simulink model "case1"  (R2024b)
settings: Solver=FixedStepAuto  StartTime=0  StopTime=1  FixedStep=1e-7  RelTol=1e-3
values from neighbouring files (symbols this model uses):
  SG_D_1_D = 0.01056    [IEEE9_case_parameters.m]    (also in case1_parameters.m; case2_parameters.m; case3_parameters.m; case4_parameters.m)
  SG_D_1_EnableSaturation = 0    [IEEE9_case_parameters.m]    (also in case1_parameters.m; case2_parameters.m; case3_parameters.m; case4_parameters.m)
  SG_D_1_f0 = 60    [IEEE9_case_parameters.m]    (also in case1_parameters.m; case2_parameters.m; case3_parameters.m; case4_parameters.m)
  SG_D_1_H = 7.5    [IEEE9_case_parameters.m]    (also in case1_parameters.m; case2_parameters.m; case3_parameters.m; case4_parameters.m)
  SG_D_1_K_A = 20    [IEEE9_case_parameters.m]    (also in case1_parameters.m; case2_parameters.m; case3_parameters.m; case4_parameters.m)
  SG_D_1_K_E = 1.000000e+1    (= 10)    [IEEE9_case_parameters.m]    (also in case1_parameters.m; case2_parameters.m; case3_parameters.m; case4_parameters.m)
  SG_D_1_K_F = 2.363    [IEEE9_case_parameters.m]    (also in case1_parameters.m; case2_parameters.m; case3_parameters.m; case4_parameters.m)
  SG_D_1_K_s = 0.5    [IEEE9_case_parameters.m]    (also in case1_parameters.m = 5; case2_parameters.m = 5; case3_parameters.m = 5; case4_parameters.m = 5)
  SG_D_1_R_a = 0.001088    [IEEE9_case_parameters.m]    (also in case1_parameters.m; case2_parameters.m; case3_parameters.m; case4_parameters.m)
  SG_D_1_S_A = 1    [IEEE9_case_parameters.m]    (also in case1_parameters.m; case2_parameters.m; case3_parameters.m; case4_parameters.m)
  SG_D_1_S_B = 0.103    [IEEE9_case_parameters.m]    (also in case1_parameters.m; case2_parameters.m; case3_parameters.m; case4_parameters.m)
  SG_D_1_S_N = 10.659857    [IEEE9_case_parameters.m]    (also in case1_parameters.m; case2_parameters.m; case3_parameters.m; case4_parameters.m)
  SG_D_1_SpeedPara = 200    [IEEE9_case_parameters.m]    (also in case1_parameters.m; case2_parameters.m; case3_parameters.m; case4_parameters.m)
  SG_D_1_T_0 = 0.720173    [IEEE9_case_parameters.m]    (also in case1_parameters.m = 0.755522; case2_parameters.m = 0.808931; case3_parameters.m = 0.869402; case4_parameters.m = 0.729316)
  SG_D_1_T_1 = 0.3    [IEEE9_case_parameters.m]    (also in case1_parameters.m; case2_parameters.m; case3_parameters.m; case4_parameters.m)
  SG_D_1_T_2 = 0.05    [IEEE9_case_parameters.m]    (also in case1_parameters.m; case2_parameters.m; case3_parameters.m; case4_parameters.m)
  SG_D_1_T_3 = 0.02    [IEEE9_case_parameters.m]    (also in case1_parameters.m; case2_parameters.m; case3_parameters.m; case4_parameters.m)
  SG_D_1_T_4 = 0.005    [IEEE9_case_parameters.m]    (also in case1_parameters.m; case2_parameters.m; case3_parameters.m; case4_parameters.m)
  SG_D_1_T_A = 0.02    [IEEE9_case_parameters.m]    (also in case1_parameters.m; case2_parameters.m; case3_parameters.m; case4_parameters.m)
  SG_D_1_T_dd = 8.000000e+0    (= 8)    [IEEE9_case_parameters.m]    (also in case1_parameters.m; case2_parameters.m; case3_parameters.m; case4_parameters.m)
  SG_D_1_T_ddd = 0.04    [IEEE9_case_parameters.m]    (also in case1_parameters.m; case2_parameters.m; case3_parameters.m; case4_parameters.m)
  SG_D_1_T_E = 0.314    [IEEE9_case_parameters.m]    (also in case1_parameters.m; case2_parameters.m; case3_parameters.m; case4_parameters.m)
  SG_D_1_T_F = 0.35    [IEEE9_case_parameters.m]    (also in case1_parameters.m; case2_parameters.m; case3_parameters.m; case4_parameters.m)
  SG_D_1_T_qd = 0.8    [IEEE9_case_parameters.m]    (also in case1_parameters.m; case2_parameters.m; case3_parameters.m; case4_parameters.m)
  SG_D_1_T_qdd = 0.02    [IEEE9_case_parameters.m]    (also in case1_parameters.m; case2_parameters.m; case3_parameters.m; case4_parameters.m)
  SG_D_1_T_speed = 0.1    [IEEE9_case_parameters.m]    (also in case1_parameters.m = 200; case2_parameters.m = 200; case3_parameters.m = 200; case4_parameters.m = 200)
  SG_D_1_T_w = 0.5    [IEEE9_case_parameters.m]    (also in case1_parameters.m; case2_parameters.m; case3_parameters.m; case4_parameters.m)
  SG_D_1_V_ref = 1.990276    [IEEE9_case_parameters.m]    (also in case1_parameters.m = 2.042296; case2_parameters.m = 2.051388; case3_parameters.m = 2.089584; case4_parameters.m = 2.01845)
  SG_D_1_w_ref = 376.991118    [IEEE9_case_parameters.m]    (also in case1_parameters.m; case2_parameters.m; case3_parameters.m; case4_parameters.m)
  SG_D_1_wb = 6.000000e+1    (= 60)    [IEEE9_case_parameters.m]    (also in case1_parameters.m; case2_parameters.m; case3_parameters.m; case4_parameters.m)
  SG_D_1_x_d = 1.9    [IEEE9_case_parameters.m]    (also in case1_parameters.m; case2_parameters.m; case3_parameters.m; case4_parameters.m)
  SG_D_1_x_dd = 0.302    [IEEE9_case_parameters.m]    (also in case1_parameters.m; case2_parameters.m; case3_parameters.m; case4_parameters.m)
  SG_D_1_x_ddd = 0.204    [IEEE9_case_parameters.m]    (also in case1_parameters.m; case2_parameters.m; case3_parameters.m; case4_parameters.m)
  SG_D_1_x_l = 0.05    [IEEE9_case_parameters.m]    (also in case1_parameters.m; case2_parameters.m; case3_parameters.m; case4_parameters.m)
  SG_D_1_x_q = 1.3    [IEEE9_case_parameters.m]    (also in case1_parameters.m; case2_parameters.m; case3_parameters.m; case4_parameters.m)
  SG_D_1_x_qd = 0.5    [IEEE9_case_parameters.m]    (also in case1_parameters.m; case2_parameters.m; case3_parameters.m; case4_parameters.m)
  SG_D_1_x_qdd = 0.3    [IEEE9_case_parameters.m]    (also in case1_parameters.m; case2_parameters.m; case3_parameters.m; case4_parameters.m)
  SG_D_2_D = 0.02    [IEEE9_case_parameters.m]    (also in case1_parameters.m; case2_parameters.m; case3_parameters.m; case4_parameters.m)
  SG_D_2_EnableSaturation = 0    [IEEE9_case_parameters.m]    (also in case1_parameters.m; case2_parameters.m; case3_parameters.m; case4_parameters.m)
  SG_D_2_f0 = 60    [IEEE9_case_parameters.m]    (also in case1_parameters.m; case2_parameters.m; case3_parameters.m; case4_parameters.m)
  SG_D_2_H = 8.000000e+0    (= 8)    [IEEE9_case_parameters.m]    (also in case1_parameters.m; case2_parameters.m; case3_parameters.m; case4_parameters.m)
  SG_D_2_K_A = 20    [IEEE9_case_parameters.m]    (also in case1_parameters.m; case2_parameters.m; case3_parameters.m; case4_parameters.m)
  SG_D_2_K_E = 1.000000e+1    (= 10)    [IEEE9_case_parameters.m]    (also in case1_parameters.m; case2_parameters.m; case3_parameters.m; case4_parameters.m)
  SG_D_2_K_F = 2.363    [IEEE9_case_parameters.m]    (also in case1_parameters.m; case2_parameters.m; case3_parameters.m; case4_parameters.m)
  SG_D_2_K_s = 0.5    [IEEE9_case_parameters.m]    (also in case1_parameters.m = 4; case2_parameters.m = 4; case3_parameters.m = 4; case4_parameters.m = 4)
  SG_D_2_R_a = 0.001088    [IEEE9_case_parameters.m]    (also in case1_parameters.m; case2_parameters.m; case3_parameters.m; case4_parameters.m)
  SG_D_2_S_A = 1    [IEEE9_case_parameters.m]    (also in case1_parameters.m; case2_parameters.m; case3_parameters.m; case4_parameters.m)
  SG_D_2_S_B = 0.103    [IEEE9_case_parameters.m]    (also in case1_parameters.m; case2_parameters.m; case3_parameters.m; case4_parameters.m)
  SG_D_2_S_N = 10.659857    [IEEE9_case_parameters.m]    (also in case1_parameters.m; case2_parameters.m; case3_parameters.m; case4_parameters.m)
  SG_D_2_SpeedPara = 200    [IEEE9_case_parameters.m]    (also in case1_parameters.m; case2_parameters.m; case3_parameters.m; case4_parameters.m)
  SG_D_2_T_0 = 1.632913    [IEEE9_case_parameters.m]    (also in case1_parameters.m = 1.632925; case2_parameters.m = 1.632915; case3_parameters.m = 1.632914; case4_parameters.m = 1.632927)
  SG_D_2_T_1 = 0.2    [IEEE9_case_parameters.m]    (also in case1_parameters.m; case2_parameters.m; case3_parameters.m; case4_parameters.m)
  SG_D_2_T_2 = 0.05    [IEEE9_case_parameters.m]    (also in case1_parameters.m; case2_parameters.m; case3_parameters.m; case4_parameters.m)
  SG_D_2_T_3 = 0.02    [IEEE9_case_parameters.m]    (also in case1_parameters.m; case2_parameters.m; case3_parameters.m; case4_parameters.m)
  SG_D_2_T_4 = 0.005    [IEEE9_case_parameters.m]    (also in case1_parameters.m; case2_parameters.m; case3_parameters.m; case4_parameters.m)
  SG_D_2_T_A = 0.02    [IEEE9_case_parameters.m]    (also in case1_parameters.m; case2_parameters.m; case3_parameters.m; case4_parameters.m)
  SG_D_2_T_dd = 7.9    [IEEE9_case_parameters.m]    (also in case1_parameters.m; case2_parameters.m; case3_parameters.m; case4_parameters.m)
  SG_D_2_T_ddd = 0.04    [IEEE9_case_parameters.m]    (also in case1_parameters.m; case2_parameters.m; case3_parameters.m; case4_parameters.m)
  SG_D_2_T_E = 0.314    [IEEE9_case_parameters.m]    (also in case1_parameters.m; case2_parameters.m; case3_parameters.m; case4_parameters.m)
  SG_D_2_T_F = 0.35    [IEEE9_case_parameters.m]    (also in case1_parameters.m; case2_parameters.m; case3_parameters.m; case4_parameters.m)
  SG_D_2_T_qd = 0.8    [IEEE9_case_parameters.m]    (also in case1_parameters.m; case2_parameters.m; case3_parameters.m; case4_parameters.m)
  SG_D_2_T_qdd = 0.015    [IEEE9_case_parameters.m]    (also in case1_parameters.m; case2_parameters.m; case3_parameters.m; case4_parameters.m)
  SG_D_2_T_speed = 0.1    [IEEE9_case_parameters.m]    (also in case1_parameters.m = 150; case2_parameters.m = 150; case3_parameters.m = 150; case4_parameters.m = 150)
  SG_D_2_T_w = 0.35    [IEEE9_case_parameters.m]    (also in case1_parameters.m; case2_parameters.m; case3_parameters.m; case4_parameters.m)
  SG_D_2_V_ref = 2.58547    [IEEE9_case_parameters.m]    (also in case1_parameters.m = 2.597896; case2_parameters.m = 2.587136; case3_parameters.m = 2.586042; case4_parameters.m = 2.599679)
  SG_D_2_w_ref = 376.991118    [IEEE9_case_parameters.m]    (also in case1_parameters.m; case2_parameters.m; case3_parameters.m; case4_parameters.m)
  SG_D_2_wb = 6.000000e+1    (= 60)    [IEEE9_case_parameters.m]    (also in case1_parameters.m; case2_parameters.m; case3_parameters.m; case4_parameters.m)
  SG_D_2_x_d = 1.8    [IEEE9_case_parameters.m]    (also in case1_parameters.m; case2_parameters.m; case3_parameters.m; case4_parameters.m)
  SG_D_2_x_dd = 0.302    [IEEE9_case_parameters.m]    (also in case1_parameters.m; case2_parameters.m; case3_parameters.m; case4_parameters.m)
  SG_D_2_x_ddd = 0.204    [IEEE9_case_parameters.m]    (also in case1_parameters.m; case2_parameters.m; case3_parameters.m; case4_parameters.m)
  SG_D_2_x_l = 0.05    [IEEE9_case_parameters.m]    (also in case1_parameters.m; case2_parameters.m; case3_parameters.m; case4_parameters.m)
  SG_D_2_x_q = 1.25    [IEEE9_case_parameters.m]    (also in case1_parameters.m; case2_parameters.m; case3_parameters.m; case4_parameters.m)
  SG_D_2_x_qd = 0.5    [IEEE9_case_parameters.m]    (also in case1_parameters.m; case2_parameters.m; case3_parameters.m; case4_parameters.m)
  SG_D_2_x_qdd = 0.3    [IEEE9_case_parameters.m]    (also in case1_parameters.m; case2_parameters.m; case3_parameters.m; case4_parameters.m)
  SG_D_3_D = 0.02    [IEEE9_case_parameters.m]    (also in case1_parameters.m; case2_parameters.m; case3_parameters.m; case4_parameters.m)
  SG_D_3_EnableSaturation = 0    [IEEE9_case_parameters.m]    (also in case1_parameters.m; case2_parameters.m; case3_parameters.m; case4_parameters.m)
  SG_D_3_f0 = 60    [IEEE9_case_parameters.m]    (also in case1_parameters.m; case2_parameters.m; case3_parameters.m; case4_parameters.m)
  SG_D_3_H = 7.7    [IEEE9_case_parameters.m]    (also in case1_parameters.m; case2_parameters.m; case3_parameters.m; case4_parameters.m)
  SG_D_3_K_A = 20    [IEEE9_case_parameters.m]    (also in case1_parameters.m; case2_parameters.m; case3_parameters.m; case4_parameters.m)
  SG_D_3_K_E = 1.000000e+1    (= 10)    [IEEE9_case_parameters.m]    (also in case1_parameters.m; case2_parameters.m; case3_parameters.m; case4_parameters.m)
  SG_D_3_K_F = 2.363    [IEEE9_case_parameters.m]    (also in case1_parameters.m; case2_parameters.m; case3_parameters.m; case4_parameters.m)
  SG_D_3_K_s = 0.2    [IEEE9_case_parameters.m]    (also in case1_parameters.m = 2; case2_parameters.m = 2; case3_parameters.m = 2; case4_parameters.m = 2)
  SG_D_3_R_a = 0.001088    [IEEE9_case_parameters.m]    (also in case1_parameters.m; case2_parameters.m; case3_parameters.m; case4_parameters.m)
  SG_D_3_S_A = 1    [IEEE9_case_parameters.m]    (also in case1_parameters.m; case2_parameters.m; case3_parameters.m; case4_parameters.m)
  SG_D_3_S_B = 0.103    [IEEE9_case_parameters.m]    (also in case1_parameters.m; case2_parameters.m; case3_parameters.m; case4_parameters.m)
  SG_D_3_S_N = 10.659857    [IEEE9_case_parameters.m]    (also in case1_parameters.m; case2_parameters.m; case3_parameters.m; case4_parameters.m)
  SG_D_3_SpeedPara = 200    [IEEE9_case_parameters.m]    (also in case1_parameters.m; case2_parameters.m; case3_parameters.m; case4_parameters.m)
  SG_D_3_T_0 = 0.850788    [IEEE9_case_parameters.m]    (also in case1_parameters.m = 0.850786; case2_parameters.m = 0.850787; case3_parameters.m; case4_parameters.m = 0.850786)
  SG_D_3_T_1 = 0.2    [IEEE9_case_parameters.m]    (also in case1_parameters.m; case2_parameters.m; case3_parameters.m; case4_parameters.m)
  SG_D_3_T_2 = 0.05    [IEEE9_case_parameters.m]    (also in case1_parameters.m; case2_parameters.m; case3_parameters.m; case4_parameters.m)
  SG_D_3_T_3 = 0.02    [IEEE9_case_parameters.m]    (also in case1_parameters.m; case2_parameters.m; case3_parameters.m; case4_parameters.m)
  SG_D_3_T_4 = 0.005    [IEEE9_case_parameters.m]    (also in case1_parameters.m; case2_parameters.m; case3_parameters.m; case4_parameters.m)
  SG_D_3_T_A = 0.02    [IEEE9_case_parameters.m]    (also in case1_parameters.m; case2_parameters.m; case3_parameters.m; case4_parameters.m)
  SG_D_3_T_dd = 8.1    [IEEE9_case_parameters.m]    (also in case1_parameters.m; case2_parameters.m; case3_parameters.m; case4_parameters.m)
  SG_D_3_T_ddd = 0.04    [IEEE9_case_parameters.m]    (also in case1_parameters.m; case2_parameters.m; case3_parameters.m; case4_parameters.m)
  SG_D_3_T_E = 0.314    [IEEE9_case_parameters.m]    (also in case1_parameters.m; case2_parameters.m; case3_parameters.m; case4_parameters.m)
  SG_D_3_T_F = 0.35    [IEEE9_case_parameters.m]    (also in case1_parameters.m; case2_parameters.m; case3_parameters.m; case4_parameters.m)
  SG_D_3_T_qd = 0.8    [IEEE9_case_parameters.m]    (also in case1_parameters.m; case2_parameters.m; case3_parameters.m; case4_parameters.m)
  SG_D_3_T_qdd = 0.015    [IEEE9_case_parameters.m]    (also in case1_parameters.m; case2_parameters.m; case3_parameters.m; case4_parameters.m)
  SG_D_3_T_speed = 0.1    [IEEE9_case_parameters.m]    (also in case1_parameters.m = 180; case2_parameters.m = 180; case3_parameters.m = 180; case4_parameters.m = 180)
  SG_D_3_T_w = 0.4    [IEEE9_case_parameters.m]    (also in case1_parameters.m; case2_parameters.m; case3_parameters.m; case4_parameters.m)
  SG_D_3_V_ref = 1.892727    [IEEE9_case_parameters.m]    (also in case1_parameters.m = 1.906439; case2_parameters.m = 1.895535; case3_parameters.m = 1.892105; case4_parameters.m = 1.906598)
  SG_D_3_w_ref = 376.991118    [IEEE9_case_parameters.m]    (also in case1_parameters.m; case2_parameters.m; case3_parameters.m; case4_parameters.m)
  SG_D_3_wb = 6.000000e+1    (= 60)    [IEEE9_case_parameters.m]    (also in case1_parameters.m; case2_parameters.m; case3_parameters.m; case4_parameters.m)
  SG_D_3_x_d = 1.85    [IEEE9_case_parameters.m]    (also in case1_parameters.m; case2_parameters.m; case3_parameters.m; case4_parameters.m)
  SG_D_3_x_dd = 0.302    [IEEE9_case_parameters.m]    (also in case1_parameters.m; case2_parameters.m; case3_parameters.m; case4_parameters.m)
  SG_D_3_x_ddd = 0.204    [IEEE9_case_parameters.m]    (also in case1_parameters.m; case2_parameters.m; case3_parameters.m; case4_parameters.m)
  SG_D_3_x_l = 0.05    [IEEE9_case_parameters.m]    (also in case1_parameters.m; case2_parameters.m; case3_parameters.m; case4_parameters.m)
  SG_D_3_x_q = 1.2    [IEEE9_case_parameters.m]    (also in case1_parameters.m; case2_parameters.m; case3_parameters.m; case4_parameters.m)
  SG_D_3_x_qd = 0.5    [IEEE9_case_parameters.m]    (also in case1_parameters.m; case2_parameters.m; case3_parameters.m; case4_parameters.m)
  SG_D_3_x_qdd = 0.3    [IEEE9_case_parameters.m]    (also in case1_parameters.m; case2_parameters.m; case3_parameters.m; case4_parameters.m)
(part 9 of 12)

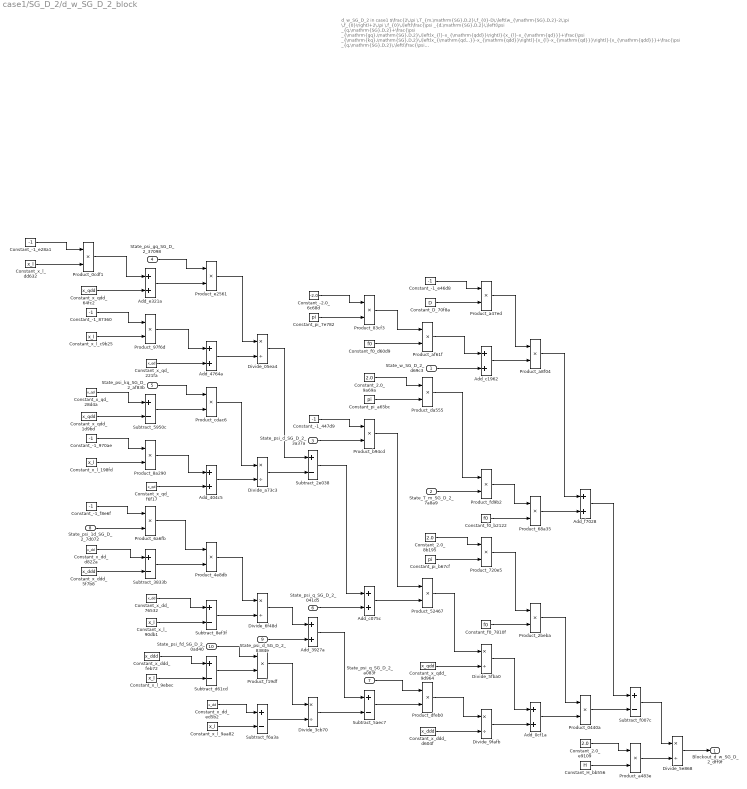
== system case1/SG_D_2/d_w_SG_D_2_block ==
  note: d_w_SG_D_2 in case1
      | $\frac{2\,\pi \,T_{m,\mathrm{SG},D,2}\,f_{0}-D\,\left(w_{\mathrm{SG},D,2}-2\,\pi \,f_{0}\right)+2\,\pi \,f_{0}\,\left(\frac{\psi _{d,\mathrm{SG},D,2}\,\left(\psi _{q,\mathrm{SG},D,2}+\frac{\psi _{\mathrm{gq},\mathrm{SG},D,2}\,\left(x_{l}-x_{\mathrm{qdd}}\right)}{x_{l}-x_{\mathrm{qd}}}+\frac{\psi _{\mathrm{kq},\mathrm{SG},D,2}\,\left(x_{\mathrm{qd}}-x_{\mathrm{qdd}}\right)}{x_{l}-x_{\mathrm{qd}}}\right)}{x_{\mathrm{qdd}}}+\frac{\psi _{q,\mathrm{SG},D,2}\,\left(\frac{\psi _{\mathrm{1d},\mathrm{SG},D,2}\,\left(x_{\mathrm{dd}}-x_{\mathrm{ddd}}\right)}{x_{\mathrm{dd}}-x_{l}}-\psi _{d,\mathrm{SG},D,2}+\frac{\psi _{\mathrm{fd},\mathrm{SG},D,2}\,\left(x_{\mathrm{ddd}}-x_{l}\right)}{x_{\mathrm{dd}}-x_{l}}\right)}{x_{\mathrm{ddd}}}\right)}{2\,H}$
      | Automatically generated on 2025-10-31 18:48:37 .
  State_w_SG_D_2_d69c3 : Inport
  State_T_m_SG_D_2_7a8a9 : Inport  Port=2
  State_psi_d_SG_D_2_3a37a : Inport  Port=3
  State_psi_gq_SG_D_2_37098 : Inport  Port=4
  State_psi_kq_SG_D_2_af83b : Inport  Port=5
  State_psi_q_SG_D_2_041d5 : Inport  Port=6
  State_psi_q_SG_D_2_a083f : Inport  Port=7
  State_psi_1d_SG_D_2_7d072 : Inport  Port=8
  State_psi_d_SG_D_2_8384e : Inport  Port=9
  State_psi_fd_SG_D_2_0ad40 : Inport  Port=10
  Add_0cf1a : Sum
  Add_3927a : Sum
  Add_404c5 : Sum
  Add_4764a : Sum
  Add_c075c : Sum
  Add_c1962 : Sum
  Add_e321a : Sum
  Add_f7028 : Sum
  Constant_-1_447d9 : Constant  Value=-1
  Constant_-1_87360 : Constant  Value=-1
  Constant_-1_970ae : Constant  Value=-1
  Constant_-1_e28a1 : Constant  Value=-1
  Constant_-1_e46d8 : Constant  Value=-1
  Constant_-1_f8e6f : Constant  Value=-1
  Constant_-2.0_6c68d : Constant  Value=-2.0
  Constant_2.0_8b195 : Constant  Value=2.0
  Constant_2.0_9a69a : Constant  Value=2.0
  Constant_2.0_e9109 : Constant  Value=2.0
  Constant_D_70f8a : Constant  Value=D
  Constant_H_bb556 : Constant  Value=H
  Constant_f0_7810f : Constant  Value=f0
  Constant_f0_b2122 : Constant  Value=f0
  Constant_f0_d60d9 : Constant  Value=f0
  Constant_pi_7e782 : Constant  Value=pi
  Constant_pi_a65bc : Constant  Value=pi
  Constant_pi_b67cf : Constant  Value=pi
  Constant_x_dd_76532 : Constant  Value=x_dd
  Constant_x_dd_d822a : Constant  Value=x_dd
  Constant_x_dd_ed5b2 : Constant  Value=x_dd
  Constant_x_ddd_5f7b8 : Constant  Value=x_ddd
  Constant_x_ddd_d604f : Constant  Value=x_ddd
  Constant_x_ddd_feb72 : Constant  Value=x_ddd
  Constant_x_l_198fd : Constant  Value=x_l
  Constant_x_l_90db1 : Constant  Value=x_l
  Constant_x_l_9aa82 : Constant  Value=x_l
  Constant_x_l_9ebec : Constant  Value=x_l
  Constant_x_l_c9b25 : Constant  Value=x_l
  Constant_x_l_dd632 : Constant  Value=x_l
  Constant_x_qd_221fa : Constant  Value=x_qd
  Constant_x_qd_28d4a : Constant  Value=x_qd
  Constant_x_qd_f6f17 : Constant  Value=x_qd
  Constant_x_qdd_1d9bd : Constant  Value=x_qdd
  Constant_x_qdd_64fc2 : Constant  Value=x_qdd
  Constant_x_qdd_9d964 : Constant  Value=x_qdd
  Divide_05ea4 : Product  Inputs=*/
  Divide_3cb70 : Product  Inputs=*/
  Divide_5e868 : Product  Inputs=*/
  Divide_5fba0 : Product  Inputs=*/
  Divide_6f48d : Product  Inputs=*/
  Divide_9fafb : Product  Inputs=*/
  Divide_a73c3 : Product  Inputs=*/
  Product_0440a : Product
  Product_0cdf1 : Product
  Product_2beba : Product
  Product_4e8db : Product
  Product_52467 : Product
  Product_68a35 : Product
  Product_6a6fb : Product
  Product_720e5 : Product
  Product_83cf3 : Product
  Product_8a290 : Product
  Product_97f6d : Product
  Product_a47ed : Product
  Product_a483e : Product
  Product_a8f04 : Product
  Product_af61f : Product
  Product_b94cd : Product
  Product_cdac6 : Product
  Product_da555 : Product
  Product_dfeb0 : Product
  Product_e2561 : Product
  Product_f19df : Product
  Product_fd9b2 : Product
  Subtract_2e038 : Sum  Inputs=+-
  Subtract_3833b : Sum  Inputs=+-
  Subtract_5950c : Sum  Inputs=+-
  Subtract_5aec7 : Sum  Inputs=+-
  Subtract_8ef3f : Sum  Inputs=+-
  Subtract_d61cd : Sum  Inputs=+-
  Subtract_f007c : Sum  Inputs=+-
  Subtract_f6a3a : Sum  Inputs=+-
  Blockout_d_w_SG_D_2_dff9f : Outport
  wires:
  Constant_x_qd_28d4a/1 -> Subtract_5950c/1
  Constant_-1_970ae/1 -> Product_8a290/1
  Constant_-1_e28a1/1 -> Product_0cdf1/1
  Constant_x_qdd_1d9bd/1 -> Subtract_5950c/2
  Subtract_f6a3a/1 -> Divide_3cb70/2
  Constant_x_l_198fd/1 -> Product_8a290/2
  Constant_x_l_dd632/1 -> Product_0cdf1/2
  Product_8a290/1 -> Add_404c5/1
  Product_0cdf1/1 -> Add_e321a/1
  Constant_x_l_90db1/1 -> Subtract_8ef3f/2
  Constant_x_l_c9b25/1 -> Product_97f6d/2
  Constant_x_ddd_d604f/1 -> Divide_9fafb/2
  Subtract_d61cd/1 -> Product_f19df/2
  Constant_x_qd_f6f17/1 -> Add_404c5/2
  Constant_x_qdd_64fc2/1 -> Add_e321a/2
  Constant_-1_87360/1 -> Product_97f6d/1
  State_psi_d_SG_D_2_3a37a/1 -> Product_b94cd/2
  Constant_-1_f8e6f/1 -> Product_6a6fb/1
  State_w_SG_D_2_d69c3/1 -> Add_c1962/2
  Product_97f6d/1 -> Add_4764a/1
  State_psi_1d_SG_D_2_7d072/1 -> Product_6a6fb/2
  Constant_x_dd_d822a/1 -> Subtract_3833b/1
  Divide_05ea4/1 -> Subtract_2e038/1
  Subtract_5950c/1 -> Product_cdac6/2
  Constant_x_ddd_5f7b8/1 -> Subtract_3833b/2
  State_psi_gq_SG_D_2_37098/1 -> Product_e2561/1
  Add_404c5/1 -> Divide_a73c3/2
  State_psi_d_SG_D_2_8384e/1 -> Add_3927a/2
  Add_e321a/1 -> Product_e2561/2
  Constant_x_qd_221fa/1 -> Add_4764a/2
  State_psi_kq_SG_D_2_af83b/1 -> Product_cdac6/1
  Product_6a6fb/1 -> Product_4e8db/1
  Subtract_3833b/1 -> Product_4e8db/2
  Constant_pi_a65bc/1 -> Product_da555/2
  Constant_x_dd_76532/1 -> Subtract_8ef3f/1
  Constant_x_ddd_feb72/1 -> Subtract_d61cd/1
  Constant_x_l_9ebec/1 -> Subtract_d61cd/2
  Product_e2561/1 -> Divide_05ea4/1
  Add_4764a/1 -> Divide_05ea4/2
  Add_c075c/1 -> Product_52467/2
  Product_cdac6/1 -> Divide_a73c3/1
  Constant_pi_7e782/1 -> Product_83cf3/2
  Product_4e8db/1 -> Divide_6f48d/1
  Subtract_8ef3f/1 -> Divide_6f48d/2
  State_psi_fd_SG_D_2_0ad40/1 -> Product_f19df/1
  Divide_6f48d/1 -> Add_3927a/1
  Constant_x_dd_ed5b2/1 -> Subtract_f6a3a/1
  Constant_x_l_9aa82/1 -> Subtract_f6a3a/2
  Divide_a73c3/1 -> Subtract_2e038/2
  Product_f19df/1 -> Divide_3cb70/1
  Constant_-1_447d9/1 -> Product_b94cd/1
  Constant_-2.0_6c68d/1 -> Product_83cf3/1
  Subtract_2e038/1 -> Add_c075c/1
  Subtract_5aec7/1 -> Product_dfeb0/2
  State_psi_q_SG_D_2_041d5/1 -> Add_c075c/2
  Constant_D_70f8a/1 -> Product_a47ed/2
  Add_3927a/1 -> Subtract_5aec7/1
  Divide_3cb70/1 -> Subtract_5aec7/2
  Product_83cf3/1 -> Product_af61f/1
  Constant_f0_d60d9/1 -> Product_af61f/2
  Constant_2.0_9a69a/1 -> Product_da555/1
  Product_b94cd/1 -> Product_52467/1
  State_psi_q_SG_D_2_a083f/1 -> Product_dfeb0/1
  Constant_-1_e46d8/1 -> Product_a47ed/1
  Product_af61f/1 -> Add_c1962/1
  Product_da555/1 -> Product_fd9b2/1
  State_T_m_SG_D_2_7a8a9/1 -> Product_fd9b2/2
  Constant_2.0_8b195/1 -> Product_720e5/1
  Constant_pi_b67cf/1 -> Product_720e5/2
  Product_52467/1 -> Divide_5fba0/1
  Constant_x_qdd_9d964/1 -> Divide_5fba0/2
  Product_dfeb0/1 -> Divide_9fafb/1
  Product_a47ed/1 -> Product_a8f04/1
  Add_c1962/1 -> Product_a8f04/2
  Product_fd9b2/1 -> Product_68a35/1
  Constant_f0_b2122/1 -> Product_68a35/2
  Product_720e5/1 -> Product_2beba/1
  Constant_f0_7810f/1 -> Product_2beba/2
  Divide_5fba0/1 -> Add_0cf1a/1
  Divide_9fafb/1 -> Add_0cf1a/2
  Product_a8f04/1 -> Add_f7028/1
  Product_68a35/1 -> Add_f7028/2
  Product_2beba/1 -> Product_0440a/1
  Add_0cf1a/1 -> Product_0440a/2
  Add_f7028/1 -> Subtract_f007c/1
  Product_0440a/1 -> Subtract_f007c/2
  Constant_2.0_e9109/1 -> Product_a483e/1
  Constant_H_bb556/1 -> Product_a483e/2
  Subtract_f007c/1 -> Divide_5e868/1
  Product_a483e/1 -> Divide_5e868/2
  Divide_5e868/1 -> Blockout_d_w_SG_D_2_dff9f/1

== system case1/SG_D_2/i_d_SG_D_2_block ==
  note: i_d_SG_D_2 in case1
      | $\frac{\sin\left(\theta _{\mathrm{SG},D,2}\right)\,\left(\frac{\psi _{\mathrm{1d},\mathrm{SG},D,2}\,\left(x_{\mathrm{dd}}-x_{\mathrm{ddd}}\right)}{x_{\mathrm{dd}}-x_{l}}-\psi _{d,\mathrm{SG},D,2}+\frac{\psi _{\mathrm{fd},\mathrm{SG},D,2}\,\left(x_{\mathrm{ddd}}-x_{l}\right)}{x_{\mathrm{dd}}-x_{l}}\right)}{x_{\mathrm{ddd}}}-\frac{\cos\left(\theta _{\mathrm{SG},D,2}\right)\,\left(\psi _{q,\mathrm{SG},D,2}+\frac{\psi _{\mathrm{gq},\mathrm{SG},D,2}\,\left(x_{l}-x_{\mathrm{qdd}}\right)}{x_{l}-x_{\mathrm{qd}}}+\frac{\psi _{\mathrm{kq},\mathrm{SG},D,2}\,\left(x_{\mathrm{qd}}-x_{\mathrm{qdd}}\right)}{x_{l}-x_{\mathrm{qd}}}\right)}{x_{\mathrm{qdd}}}$
      | Automatically generated on 2025-10-31 18:49:00 .
  State_psi_gq_SG_D_2_0a4ff : Inport
  State_psi_kq_SG_D_2_7acfc : Inport  Port=2
  State_psi_q_SG_D_2_a8ffe : Inport  Port=3
  State_theta_SG_D_2_c8d9f : Inport  Port=4
  State_psi_1d_SG_D_2_a6845 : Inport  Port=5
  State_psi_d_SG_D_2_bb259 : Inport  Port=6
  State_psi_fd_SG_D_2_62171 : Inport  Port=7
  State_theta_SG_D_2_f5053 : Inport  Port=8
  Add_011cd : Sum
  Add_0850a : Sum
  Add_a0ac0 : Sum
  Add_dc8be : Sum
  Add_f42b2 : Sum
  Constant_-1_0c488 : Constant  Value=-1
  Constant_-1_0f0de : Constant  Value=-1
  Constant_-1_1cc01 : Constant  Value=-1
  Constant_-1_5980f : Constant  Value=-1
  Constant_-1_d33fc : Constant  Value=-1
  Constant_x_dd_00768 : Constant  Value=x_dd
  Constant_x_dd_10395 : Constant  Value=x_dd
  Constant_x_dd_b8d2d : Constant  Value=x_dd
  Constant_x_ddd_1b8f0 : Constant  Value=x_ddd
  Constant_x_ddd_22ecc : Constant  Value=x_ddd
  Constant_x_ddd_e4a9f : Constant  Value=x_ddd
  Constant_x_l_085c2 : Constant  Value=x_l
  Constant_x_l_12cb4 : Constant  Value=x_l
  Constant_x_l_79920 : Constant  Value=x_l
  Constant_x_l_95991 : Constant  Value=x_l
  Constant_x_l_a4458 : Constant  Value=x_l
  Constant_x_l_b7955 : Constant  Value=x_l
  Constant_x_qd_723dd : Constant  Value=x_qd
  Constant_x_qd_76317 : Constant  Value=x_qd
  Constant_x_qd_f66d9 : Constant  Value=x_qd
  Constant_x_qdd_28160 : Constant  Value=x_qdd
  Constant_x_qdd_83bfb : Constant  Value=x_qdd
  Constant_x_qdd_9bcae : Constant  Value=x_qdd
  Divide_3503f : Product  Inputs=*/
  Divide_4d07a : Product  Inputs=*/
  Divide_803bf : Product  Inputs=*/
  Divide_94b5e : Product  Inputs=*/
  Divide_dbe3d : Product  Inputs=*/
  Divide_e5f2f : Product  Inputs=*/
  MathFunc_cos_5ce99 : Trigonometry  Operator=cos
  MathFunc_sin_c738e : Trigonometry
  Product_0ac03 : Product
  Product_18786 : Product
  Product_2a085 : Product
  Product_752ca : Product
  Product_7ed47 : Product
  Product_88b7a : Product
  Product_91a9f : Product
  Product_a2b3c : Product
  Product_bdf87 : Product
  Product_e301a : Product
  Product_e88dc : Product
  Subtract_10957 : Sum  Inputs=+-
  Subtract_14973 : Sum  Inputs=+-
  Subtract_2a698 : Sum  Inputs=+-
  Subtract_4108c : Sum  Inputs=+-
  Subtract_8999b : Sum  Inputs=+-
  Subtract_9696a : Sum  Inputs=+-
  Subtract_a9296 : Sum  Inputs=+-
  Subtract_e7b67 : Sum  Inputs=+-
  Blockout_i_d_SG_D_2_76c8b : Outport
  wires:
  Constant_x_ddd_e4a9f/1 -> Subtract_4108c/1
  Constant_x_qd_76317/1 -> Subtract_9696a/1
  Constant_-1_0f0de/1 -> Product_0ac03/1
  Constant_-1_1cc01/1 -> Product_91a9f/1
  Subtract_10957/1 -> Blockout_i_d_SG_D_2_76c8b/1
  Constant_x_qdd_28160/1 -> Subtract_9696a/2
  Constant_x_l_085c2/1 -> Product_0ac03/2
  Constant_x_l_12cb4/1 -> Product_91a9f/2
  Product_0ac03/1 -> Add_f42b2/1
  Product_91a9f/1 -> Add_011cd/1
  Constant_x_l_95991/1 -> Product_a2b3c/2
  Constant_x_qd_723dd/1 -> Add_f42b2/2
  Constant_x_qdd_9bcae/1 -> Add_011cd/2
  Constant_x_qdd_83bfb/1 -> Divide_e5f2f/2
  MathFunc_cos_5ce99/1 -> Product_e88dc/2
  Constant_-1_5980f/1 -> Product_a2b3c/1
  State_psi_gq_SG_D_2_0a4ff/1 -> Product_88b7a/1
  Subtract_4108c/1 -> Product_7ed47/2
  Product_752ca/1 -> Product_bdf87/1
  Add_f42b2/1 -> Divide_94b5e/2
  Add_011cd/1 -> Product_88b7a/2
  Product_7ed47/1 -> Divide_dbe3d/1
  Product_a2b3c/1 -> Add_0850a/1
  Constant_x_qd_f66d9/1 -> Add_0850a/2
  State_theta_SG_D_2_f5053/1 -> MathFunc_sin_c738e/1
  State_psi_kq_SG_D_2_7acfc/1 -> Product_e301a/1
  Add_a0ac0/1 -> Subtract_14973/1
  Subtract_9696a/1 -> Product_e301a/2
  Product_88b7a/1 -> Divide_803bf/1
  Constant_-1_d33fc/1 -> Product_752ca/1
  State_psi_1d_SG_D_2_a6845/1 -> Product_752ca/2
  State_psi_fd_SG_D_2_62171/1 -> Product_7ed47/1
  Constant_x_dd_b8d2d/1 -> Subtract_e7b67/1
  Product_bdf87/1 -> Divide_3503f/1
  Constant_x_ddd_1b8f0/1 -> Subtract_e7b67/2
  Divide_dbe3d/1 -> Subtract_14973/2
  Add_0850a/1 -> Divide_803bf/2
  Product_2a085/1 -> Divide_4d07a/1
  Product_e301a/1 -> Divide_94b5e/1
  Constant_-1_0c488/1 -> Product_18786/1
  Subtract_2a698/1 -> Divide_dbe3d/2
  Subtract_e7b67/1 -> Product_bdf87/2
  Constant_x_dd_10395/1 -> Subtract_a9296/1
  Subtract_14973/1 -> Product_2a085/1
  Constant_x_l_a4458/1 -> Subtract_a9296/2
  Constant_x_l_79920/1 -> Subtract_4108c/2
  Divide_803bf/1 -> Subtract_8999b/1
  Divide_4d07a/1 -> Subtract_10957/2
  Divide_94b5e/1 -> Subtract_8999b/2
  Subtract_a9296/1 -> Divide_3503f/2
  Constant_x_dd_00768/1 -> Subtract_2a698/1
  Divide_e5f2f/1 -> Subtract_10957/1
  Constant_x_l_b7955/1 -> Subtract_2a698/2
  Subtract_8999b/1 -> Add_dc8be/1
  State_psi_q_SG_D_2_a8ffe/1 -> Add_dc8be/2
  Constant_x_ddd_22ecc/1 -> Divide_4d07a/2
  MathFunc_sin_c738e/1 -> Product_2a085/2
  Divide_3503f/1 -> Add_a0ac0/1
  State_psi_d_SG_D_2_bb259/1 -> Add_a0ac0/2
  Add_dc8be/1 -> Product_18786/2
  State_theta_SG_D_2_c8d9f/1 -> MathFunc_cos_5ce99/1
  Product_18786/1 -> Product_e88dc/1
  Product_e88dc/1 -> Divide_e5f2f/1

== system case1/SG_D_2/i_q_SG_D_2_block ==
  note: i_q_SG_D_2 in case1
      | $-\frac{\sin\left(\theta _{\mathrm{SG},D,2}\right)\,\left(\psi _{q,\mathrm{SG},D,2}+\frac{\psi _{\mathrm{gq},\mathrm{SG},D,2}\,\left(x_{l}-x_{\mathrm{qdd}}\right)}{x_{l}-x_{\mathrm{qd}}}+\frac{\psi _{\mathrm{kq},\mathrm{SG},D,2}\,\left(x_{\mathrm{qd}}-x_{\mathrm{qdd}}\right)}{x_{l}-x_{\mathrm{qd}}}\right)}{x_{\mathrm{qdd}}}-\frac{\cos\left(\theta _{\mathrm{SG},D,2}\right)\,\left(\frac{\psi _{\mathrm{1d},\mathrm{SG},D,2}\,\left(x_{\mathrm{dd}}-x_{\mathrm{ddd}}\right)}{x_{\mathrm{dd}}-x_{l}}-\psi _{d,\mathrm{SG},D,2}+\frac{\psi _{\mathrm{fd},\mathrm{SG},D,2}\,\left(x_{\mathrm{ddd}}-x_{l}\right)}{x_{\mathrm{dd}}-x_{l}}\right)}{x_{\mathrm{ddd}}}$
      | Automatically generated on 2025-10-31 18:49:05 .
  State_psi_gq_SG_D_2_4b38b : Inport
  State_psi_kq_SG_D_2_d6d60 : Inport  Port=2
  State_psi_q_SG_D_2_008e1 : Inport  Port=3
  State_theta_SG_D_2_18eff : Inport  Port=4
  State_psi_1d_SG_D_2_4cf3f : Inport  Port=5
  State_psi_d_SG_D_2_91eea : Inport  Port=6
  State_psi_fd_SG_D_2_0701d : Inport  Port=7
  State_theta_SG_D_2_18733 : Inport  Port=8
  Add_5ca14 : Sum
  Add_6d82a : Sum
  Add_6f44e : Sum
  Add_e9056 : Sum
  Add_f4be1 : Sum
  Add_f59d6 : Sum
  Constant_-1_40a27 : Constant  Value=-1
  Constant_-1_57f63 : Constant  Value=-1
  Constant_-1_6b4ac : Constant  Value=-1
  Constant_-1_817d1 : Constant  Value=-1
  Constant_-1_ca257 : Constant  Value=-1
  Constant_x_dd_6fb7b : Constant  Value=x_dd
  Constant_x_dd_e448e : Constant  Value=x_dd
  Constant_x_dd_fe1f7 : Constant  Value=x_dd
  Constant_x_ddd_28940 : Constant  Value=x_ddd
  Constant_x_ddd_6f407 : Constant  Value=x_ddd
  Constant_x_ddd_fb49d : Constant  Value=x_ddd
  Constant_x_l_24c0c : Constant  Value=x_l
  Constant_x_l_2e309 : Constant  Value=x_l
  Constant_x_l_5bf1e : Constant  Value=x_l
  Constant_x_l_67dcf : Constant  Value=x_l
  Constant_x_l_892c3 : Constant  Value=x_l
  Constant_x_l_fb301 : Constant  Value=x_l
  Constant_x_qd_7a527 : Constant  Value=x_qd
  Constant_x_qd_ba7df : Constant  Value=x_qd
  Constant_x_qd_f0477 : Constant  Value=x_qd
  Constant_x_qdd_28d4f : Constant  Value=x_qdd
  Constant_x_qdd_42422 : Constant  Value=x_qdd
  Constant_x_qdd_5bb10 : Constant  Value=x_qdd
  Divide_3d113 : Product  Inputs=*/
  Divide_3f788 : Product  Inputs=*/
  Divide_3fc0a : Product  Inputs=*/
  Divide_5492a : Product  Inputs=*/
  Divide_b503b : Product  Inputs=*/
  Divide_f7bc0 : Product  Inputs=*/
  MathFunc_cos_52f4e : Trigonometry  Operator=cos
  MathFunc_sin_22d7a : Trigonometry
  Product_3ad89 : Product
  Product_41e46 : Product
  Product_45dcf : Product
  Product_4ce7c : Product
  Product_5f6d3 : Product
  Product_6675f : Product
  Product_76c1d : Product
  Product_c3344 : Product
  Product_d360f : Product
  Product_e5525 : Product
  Product_edea1 : Product
  Subtract_0b5bd : Sum  Inputs=+-
  Subtract_2e199 : Sum  Inputs=+-
  Subtract_2ff29 : Sum  Inputs=+-
  Subtract_40cd8 : Sum  Inputs=+-
  Subtract_d5ae3 : Sum  Inputs=+-
  Subtract_df5e3 : Sum  Inputs=+-
  Subtract_f6fe2 : Sum  Inputs=+-
  Blockout_i_q_SG_D_2_02eb4 : Outport
  wires:
  MathFunc_sin_22d7a/1 -> Product_3ad89/2
  Product_45dcf/1 -> Product_3ad89/1
  Constant_-1_ca257/1 -> Product_d360f/1
  Constant_-1_6b4ac/1 -> Product_e5525/1
  Constant_x_l_2e309/1 -> Product_d360f/2
  Product_d360f/1 -> Add_f4be1/1
  Subtract_2e199/1 -> Product_5f6d3/2
  Constant_x_qdd_5bb10/1 -> Subtract_d5ae3/2
  Constant_x_qdd_28d4f/1 -> Add_f4be1/2
  Add_e9056/1 -> Product_45dcf/2
  Constant_x_l_24c0c/1 -> Product_e5525/2
  Constant_x_qd_ba7df/1 -> Subtract_d5ae3/1
  Constant_-1_817d1/1 -> Product_4ce7c/1
  Constant_x_l_67dcf/1 -> Product_4ce7c/2
  State_psi_1d_SG_D_2_4cf3f/1 -> Product_41e46/2
  State_psi_gq_SG_D_2_4b38b/1 -> Product_76c1d/1
  Add_f4be1/1 -> Product_76c1d/2
  Product_e5525/1 -> Add_5ca14/1
  Divide_b503b/1 -> Add_6d82a/1
  Constant_x_qd_7a527/1 -> Add_5ca14/2
  State_psi_kq_SG_D_2_d6d60/1 -> Product_6675f/1
  Add_6f44e/1 -> Subtract_40cd8/1
  Constant_x_ddd_6f407/1 -> Subtract_2e199/2
  Subtract_d5ae3/1 -> Product_6675f/2
  Product_4ce7c/1 -> Add_f59d6/1
  Constant_x_qd_f0477/1 -> Add_f59d6/2
  Constant_-1_40a27/1 -> Product_41e46/1
  Constant_x_l_fb301/1 -> Subtract_2ff29/2
  Constant_x_dd_6fb7b/1 -> Subtract_2e199/1
  Product_76c1d/1 -> Divide_3f788/1
  Divide_f7bc0/1 -> Subtract_40cd8/2
  Add_5ca14/1 -> Divide_3f788/2
  Product_c3344/1 -> Divide_5492a/1
  Product_6675f/1 -> Divide_3d113/1
  Constant_-1_57f63/1 -> Product_45dcf/1
  Product_41e46/1 -> Product_5f6d3/1
  Add_f59d6/1 -> Divide_3d113/2
  Constant_x_dd_e448e/1 -> Subtract_df5e3/1
  Subtract_40cd8/1 -> Product_c3344/1
  Subtract_0b5bd/1 -> Product_edea1/2
  Constant_x_l_892c3/1 -> Subtract_df5e3/2
  Constant_x_ddd_28940/1 -> Subtract_0b5bd/1
  Constant_x_l_5bf1e/1 -> Subtract_0b5bd/2
  Divide_3f788/1 -> Subtract_f6fe2/1
  Divide_5492a/1 -> Add_6d82a/2
  Product_edea1/1 -> Divide_f7bc0/1
  Divide_3d113/1 -> Subtract_f6fe2/2
  Subtract_2ff29/1 -> Divide_f7bc0/2
  Product_5f6d3/1 -> Divide_3fc0a/1
  Subtract_df5e3/1 -> Divide_3fc0a/2
  Constant_x_qdd_42422/1 -> Divide_b503b/2
  State_psi_fd_SG_D_2_0701d/1 -> Product_edea1/1
  Constant_x_dd_fe1f7/1 -> Subtract_2ff29/1
  Subtract_f6fe2/1 -> Add_e9056/1
  State_psi_q_SG_D_2_008e1/1 -> Add_e9056/2
  Constant_x_ddd_fb49d/1 -> Divide_5492a/2
  Divide_3fc0a/1 -> Add_6f44e/1
  State_psi_d_SG_D_2_91eea/1 -> Add_6f44e/2
  State_theta_SG_D_2_18eff/1 -> MathFunc_sin_22d7a/1
  State_theta_SG_D_2_18733/1 -> MathFunc_cos_52f4e/1
  MathFunc_cos_52f4e/1 -> Product_c3344/2
  Product_3ad89/1 -> Divide_b503b/1
  Add_6d82a/1 -> Blockout_i_q_SG_D_2_02eb4/1

== system case1/SG_D_2/theta_SG_D_2_out_block ==
  note: theta_SG_D_2_out in case1
      | $\theta _{\mathrm{SG},D,2}$
      | Automatically generated on 2025-10-31 18:49:10 .
  State_theta_SG_D_2_2515d : Inport
  Blockout_theta_SG_D_2_out_503d1 : Outport
  wires:
  State_theta_SG_D_2_2515d/1 -> Blockout_theta_SG_D_2_out_503d1/1

== system case1/SG_D_2/w_SG_D_2_out_block ==
  note: w_SG_D_2_out in case1
      | $w_{\mathrm{SG},D,2}$
      | Automatically generated on 2025-10-31 18:49:10 .
  State_w_SG_D_2_39d84 : Inport
  Blockout_w_SG_D_2_out_2e2ba : Outport
  wires:
  State_w_SG_D_2_39d84/1 -> Blockout_w_SG_D_2_out_2e2ba/1

== system case1/SG_D_3/T_e_SG_D_3_block ==
  note: T_e_SG_D_3 in case1
      | $-\frac{\psi _{d,\mathrm{SG},D,3}\,\left(\psi _{q,\mathrm{SG},D,3}+\frac{\psi _{\mathrm{gq},\mathrm{SG},D,3}\,\left(x_{l}-x_{\mathrm{qdd}}\right)}{x_{l}-x_{\mathrm{qd}}}+\frac{\psi _{\mathrm{kq},\mathrm{SG},D,3}\,\left(x_{\mathrm{qd}}-x_{\mathrm{qdd}}\right)}{x_{l}-x_{\mathrm{qd}}}\right)}{x_{\mathrm{qdd}}}-\frac{\psi _{q,\mathrm{SG},D,3}\,\left(\frac{\psi _{\mathrm{1d},\mathrm{SG},D,3}\,\left(x_{\mathrm{dd}}-x_{\mathrm{ddd}}\right)}{x_{\mathrm{dd}}-x_{l}}-\psi _{d,\mathrm{SG},D,3}+\frac{\psi _{\mathrm{fd},\mathrm{SG},D,3}\,\left(x_{\mathrm{ddd}}-x_{l}\right)}{x_{\mathrm{dd}}-x_{l}}\right)}{x_{\mathrm{ddd}}}$
      | Automatically generated on 2025-10-31 18:50:09 .
  State_psi_d_SG_D_3_e2290 : Inport
  State_psi_gq_SG_D_3_86cef : Inport  Port=2
  State_psi_kq_SG_D_3_cb0a5 : Inport  Port=3
  State_psi_q_SG_D_3_ebc14 : Inport  Port=4
  State_psi_q_SG_D_3_fe94c : Inport  Port=5
  State_psi_1d_SG_D_3_b91a5 : Inport  Port=6
  State_psi_d_SG_D_3_4b90d : Inport  Port=7
  State_psi_fd_SG_D_3_9749b : Inport  Port=8
  Add_251f7 : Sum
  Add_35f60 : Sum
  Add_499f6 : Sum
  Add_4e78f : Sum
  Add_cc6c9 : Sum
  Add_e5e25 : Sum
  Constant_-1_4929b : Constant  Value=-1
  Constant_-1_62150 : Constant  Value=-1
  Constant_-1_d3bf6 : Constant  Value=-1
  Constant_-1_df9b5 : Constant  Value=-1
  Constant_-1_edb41 : Constant  Value=-1
  Constant_x_dd_3daa4 : Constant  Value=x_dd
  Constant_x_dd_6c13d : Constant  Value=x_dd
  Constant_x_dd_83da4 : Constant  Value=x_dd
  Constant_x_ddd_0dccd : Constant  Value=x_ddd
  Constant_x_ddd_9734c : Constant  Value=x_ddd
  Constant_x_ddd_c98a5 : Constant  Value=x_ddd
  Constant_x_l_09a43 : Constant  Value=x_l
  Constant_x_l_4cf60 : Constant  Value=x_l
  Constant_x_l_655d4 : Constant  Value=x_l
  Constant_x_l_8810e : Constant  Value=x_l
  Constant_x_l_8ec4d : Constant  Value=x_l
  Constant_x_l_9ab7e : Constant  Value=x_l
  Constant_x_qd_a0800 : Constant  Value=x_qd
  Constant_x_qd_aa451 : Constant  Value=x_qd
  Constant_x_qd_c3d70 : Constant  Value=x_qd
  Constant_x_qdd_00d46 : Constant  Value=x_qdd
  Constant_x_qdd_3b8f5 : Constant  Value=x_qdd
  Constant_x_qdd_ebed0 : Constant  Value=x_qdd
  Divide_27cee : Product  Inputs=*/
  Divide_53822 : Product  Inputs=*/
  Divide_7f8a3 : Product  Inputs=*/
  Divide_c001f : Product  Inputs=*/
  Divide_e08b3 : Product  Inputs=*/
  Divide_ef535 : Product  Inputs=*/
  Product_1345a : Product
  Product_3ae3a : Product
  Product_46020 : Product
  Product_78035 : Product
  Product_7beb8 : Product
  Product_92909 : Product
  Product_aec94 : Product
  Product_c497d : Product
  Product_d1daa : Product
  Product_da0fb : Product
  Product_e81f8 : Product
  Subtract_1551d : Sum  Inputs=+-
  Subtract_37dc1 : Sum  Inputs=+-
  Subtract_3efda : Sum  Inputs=+-
  Subtract_42cb7 : Sum  Inputs=+-
  Subtract_a8a5c : Sum  Inputs=+-
  Subtract_bddf2 : Sum  Inputs=+-
  Subtract_d21b7 : Sum  Inputs=+-
  Blockout_T_e_SG_D_3_5971a : Outport
  wires:
  State_psi_q_SG_D_3_ebc14/1 -> Add_cc6c9/2
  Constant_-1_edb41/1 -> Product_3ae3a/1
  Subtract_a8a5c/1 -> Product_da0fb/2
  State_psi_1d_SG_D_3_b91a5/1 -> Product_1345a/2
  Constant_-1_62150/1 -> Product_7beb8/1
  Constant_x_l_09a43/1 -> Product_7beb8/2
  Add_35f60/1 -> Subtract_a8a5c/1
  State_psi_d_SG_D_3_4b90d/1 -> Add_35f60/2
  Product_7beb8/1 -> Add_499f6/1
  Constant_x_qdd_00d46/1 -> Subtract_37dc1/2
  Add_cc6c9/1 -> Product_d1daa/2
  Constant_x_qdd_3b8f5/1 -> Add_499f6/2
  State_psi_q_SG_D_3_fe94c/1 -> Product_da0fb/1
  Constant_x_l_655d4/1 -> Product_3ae3a/2
  Subtract_d21b7/1 -> Divide_53822/2
  Constant_x_l_8ec4d/1 -> Subtract_1551d/2
  Constant_x_qd_c3d70/1 -> Subtract_37dc1/1
  Constant_-1_df9b5/1 -> Product_78035/1
  Subtract_bddf2/1 -> Divide_27cee/2
  Constant_x_l_8810e/1 -> Product_78035/2
  Product_aec94/1 -> Divide_27cee/1
  Constant_-1_d3bf6/1 -> Product_1345a/1
  Product_1345a/1 -> Product_aec94/1
  Constant_x_dd_6c13d/1 -> Subtract_42cb7/1
  Constant_x_ddd_c98a5/1 -> Subtract_42cb7/2
  Add_4e78f/1 -> Blockout_T_e_SG_D_3_5971a/1
  State_psi_gq_SG_D_3_86cef/1 -> Product_c497d/1
  Product_da0fb/1 -> Divide_ef535/1
  Add_499f6/1 -> Product_c497d/2
  State_psi_fd_SG_D_3_9749b/1 -> Product_e81f8/1
  Product_3ae3a/1 -> Add_251f7/1
  Constant_x_qd_aa451/1 -> Add_251f7/2
  Constant_x_dd_83da4/1 -> Subtract_bddf2/1
  State_psi_kq_SG_D_3_cb0a5/1 -> Product_46020/1
  Constant_x_dd_3daa4/1 -> Subtract_d21b7/1
  Subtract_37dc1/1 -> Product_46020/2
  Product_d1daa/1 -> Divide_c001f/1
  Product_78035/1 -> Add_e5e25/1
  Add_251f7/1 -> Divide_7f8a3/2
  Constant_x_qd_a0800/1 -> Add_e5e25/2
  Subtract_42cb7/1 -> Product_aec94/2
  Constant_x_l_9ab7e/1 -> Subtract_bddf2/2
  Constant_x_ddd_9734c/1 -> Subtract_1551d/1
  Product_c497d/1 -> Divide_7f8a3/1
  Product_46020/1 -> Divide_e08b3/1
  Add_e5e25/1 -> Divide_e08b3/2
  Constant_x_ddd_0dccd/1 -> Divide_ef535/2
  Subtract_1551d/1 -> Product_e81f8/2
  Divide_7f8a3/1 -> Subtract_3efda/1
  Constant_x_l_4cf60/1 -> Subtract_d21b7/2
  Divide_e08b3/1 -> Subtract_3efda/2
  Divide_27cee/1 -> Add_35f60/1
  Product_e81f8/1 -> Divide_53822/1
  Constant_-1_4929b/1 -> Product_92909/1
  State_psi_d_SG_D_3_e2290/1 -> Product_92909/2
  Subtract_3efda/1 -> Add_cc6c9/1
  Divide_53822/1 -> Subtract_a8a5c/2
  Product_92909/1 -> Product_d1daa/1
  Constant_x_qdd_ebed0/1 -> Divide_c001f/2
  Divide_c001f/1 -> Add_4e78f/1
  Divide_ef535/1 -> Add_4e78f/2

== system case1/SG_D_3/d_E_fd_SG_D_3_block ==
  note: d_E_fd_SG_D_3 in case1
      | $\frac{V_{f,\mathrm{SG},D,3}-E_{\mathrm{fd},\mathrm{SG},D,3}\,K_{E}}{T_{E}}$
      | Automatically generated on 2025-10-31 18:49:57 .
  State_E_fd_SG_D_3_b50ae : Inport
  State_V_f_SG_D_3_378e4 : Inport  Port=2
  Add_15844 : Sum
  Constant_-1_9b083 : Constant  Value=-1
  Constant_K_E_ef23c : Constant  Value=K_E
  Constant_T_E_f2f88 : Constant  Value=T_E
  Divide_97146 : Product  Inputs=*/
  Product_af7b3 : Product
  Product_e4424 : Product
  Blockout_d_E_fd_SG_D_3_6f2ed : Outport
  wires:
  State_V_f_SG_D_3_378e4/1 -> Add_15844/2
  Constant_-1_9b083/1 -> Product_af7b3/1
  State_E_fd_SG_D_3_b50ae/1 -> Product_af7b3/2
  Constant_T_E_f2f88/1 -> Divide_97146/2
  Product_af7b3/1 -> Product_e4424/1
  Product_e4424/1 -> Add_15844/1
  Constant_K_E_ef23c/1 -> Product_e4424/2
  Divide_97146/1 -> Blockout_d_E_fd_SG_D_3_6f2ed/1
  Add_15844/1 -> Divide_97146/1

== system case1/SG_D_3/d_Px_1_SG_D_3_block ==
  note: d_Px_1_SG_D_3 in case1
      | $\frac{w_{\mathrm{SG},D,3}-2\,\pi \,f_{0}}{T_{w}}-\frac{\mathrm{Px}_{1,\mathrm{SG},D,3}}{T_{w}}$
      | Automatically generated on 2025-10-31 18:49:57 .
  State_Px_1_SG_D_3_d0b1d : Inport
  State_w_SG_D_3_e1b7a : Inport  Port=2
  Add_bf0f5 : Sum
  Add_c1dec : Sum
  Constant_-1_3d4ee : Constant  Value=-1
  Constant_-2.0_6ac50 : Constant  Value=-2.0
  Constant_T_w_604f9 : Constant  Value=T_w
  Constant_T_w_ad7c9 : Constant  Value=T_w
  Constant_f0_cd00b : Constant  Value=f0
  Constant_pi_59f91 : Constant  Value=pi
  Divide_00343 : Product  Inputs=*/
  Divide_de06c : Product  Inputs=*/
  Product_6bb60 : Product
  Product_d6906 : Product
  Product_f9503 : Product
  Blockout_d_Px_1_SG_D_3_617e0 : Outport
  wires:
  Constant_f0_cd00b/1 -> Product_6bb60/2
  Constant_-1_3d4ee/1 -> Product_d6906/1
  Constant_-2.0_6ac50/1 -> Product_f9503/1
  Constant_pi_59f91/1 -> Product_f9503/2
  Product_f9503/1 -> Product_6bb60/1
  State_w_SG_D_3_e1b7a/1 -> Add_bf0f5/2
  Divide_00343/1 -> Add_c1dec/1
  State_Px_1_SG_D_3_d0b1d/1 -> Product_d6906/2
  Product_6bb60/1 -> Add_bf0f5/1
  Product_d6906/1 -> Divide_00343/1
  Constant_T_w_604f9/1 -> Divide_00343/2
  Add_bf0f5/1 -> Divide_de06c/1
  Constant_T_w_ad7c9/1 -> Divide_de06c/2
  Divide_de06c/1 -> Add_c1dec/2
  Add_c1dec/1 -> Blockout_d_Px_1_SG_D_3_617e0/1

== system case1/SG_D_3/d_Px_2_SG_D_3_block ==
  note: d_Px_2_SG_D_3 in case1
      | $\frac{\mathrm{Px}_{1,\mathrm{SG},D,3}-T_{2}\,\left(\frac{\mathrm{Px}_{1,\mathrm{SG},D,3}}{T_{w}}-\frac{w_{\mathrm{SG},D,3}-2\,\pi \,f_{0}}{T_{w}}\right)}{T_{1}}-\frac{\mathrm{Px}_{2,\mathrm{SG},D,3}}{T_{1}}$
      | Automatically generated on 2025-10-31 18:49:58 .
  State_Px_2_SG_D_3_42098 : Inport
  State_Px_1_SG_D_3_f2f90 : Inport  Port=2
  State_Px_1_SG_D_3_ad022 : Inport  Port=3
  State_w_SG_D_3_b1950 : Inport  Port=4
  Add_391ba : Sum
  Add_9975d : Sum
  Add_a1d31 : Sum
  Add_eca2e : Sum
  Constant_-1_0b6a9 : Constant  Value=-1
  Constant_-1_d562d : Constant  Value=-1
  Constant_-2.0_d3c50 : Constant  Value=-2.0
  Constant_T_1_4a23a : Constant  Value=T_1
  Constant_T_1_d55d9 : Constant  Value=T_1
  Constant_T_2_56e9b : Constant  Value=T_2
  Constant_T_w_ca482 : Constant  Value=T_w
  Constant_T_w_f2583 : Constant  Value=T_w
  Constant_f0_cda18 : Constant  Value=f0
  Constant_pi_910ea : Constant  Value=pi
  Divide_20721 : Product  Inputs=*/
  Divide_22bcf : Product  Inputs=*/
  Divide_54385 : Product  Inputs=*/
  Divide_73995 : Product  Inputs=*/
  Product_4e61b : Product
  Product_76a57 : Product
  Product_d7539 : Product
  Product_e47e8 : Product
  Product_f567e : Product
  Blockout_d_Px_2_SG_D_3_63947 : Outport
  wires:
  State_Px_1_SG_D_3_ad022/1 -> Product_76a57/2
  Constant_-2.0_d3c50/1 -> Product_4e61b/1
  Constant_f0_cda18/1 -> Product_d7539/2
  Constant_pi_910ea/1 -> Product_4e61b/2
  Product_4e61b/1 -> Product_d7539/1
  State_w_SG_D_3_b1950/1 -> Add_eca2e/2
  Constant_-1_0b6a9/1 -> Product_76a57/1
  Product_d7539/1 -> Add_eca2e/1
  Product_76a57/1 -> Divide_22bcf/1
  Constant_T_w_ca482/1 -> Divide_22bcf/2
  Add_eca2e/1 -> Divide_20721/1
  Constant_T_w_f2583/1 -> Divide_20721/2
  Divide_22bcf/1 -> Add_391ba/1
  Divide_20721/1 -> Add_391ba/2
  Constant_T_2_56e9b/1 -> Product_e47e8/1
  Add_391ba/1 -> Product_e47e8/2
  Constant_-1_d562d/1 -> Product_f567e/1
  Product_e47e8/1 -> Add_a1d31/2
  State_Px_2_SG_D_3_42098/1 -> Product_f567e/2
  State_Px_1_SG_D_3_f2f90/1 -> Add_a1d31/1
  Product_f567e/1 -> Divide_54385/1
  Add_9975d/1 -> Blockout_d_Px_2_SG_D_3_63947/1
  Constant_T_1_4a23a/1 -> Divide_54385/2
  Add_a1d31/1 -> Divide_73995/1
  Constant_T_1_d55d9/1 -> Divide_73995/2
  Divide_54385/1 -> Add_9975d/1
  Divide_73995/1 -> Add_9975d/2

== system case1/SG_D_3/d_Px_3_SG_D_3_block ==
  note: d_Px_3_SG_D_3 in case1
      | $\frac{\mathrm{Px}_{2,\mathrm{SG},D,3}+T_{4}\,\left(\frac{\mathrm{Px}_{1,\mathrm{SG},D,3}-T_{2}\,\left(\frac{\mathrm{Px}_{1,\mathrm{SG},D,3}}{T_{w}}-\frac{w_{\mathrm{SG},D,3}-2\,\pi \,f_{0}}{T_{w}}\right)}{T_{1}}-\frac{\mathrm{Px}_{2,\mathrm{SG},D,3}}{T_{1}}\right)}{T_{3}}-\frac{\mathrm{Px}_{3,\mathrm{SG},D,3}}{T_{3}}$
      | Automatically generated on 2025-10-31 18:49:59 .
  State_Px_3_SG_D_3_e3475 : Inport
  State_Px_2_SG_D_3_9be0b : Inport  Port=2
  State_Px_2_SG_D_3_dd0dd : Inport  Port=3
  State_Px_1_SG_D_3_57193 : Inport  Port=4
  State_Px_1_SG_D_3_ac5bc : Inport  Port=5
  State_w_SG_D_3_60df7 : Inport  Port=6
  Add_3441e : Sum
  Add_36bb7 : Sum
  Add_4f5a0 : Sum
  Add_66dd9 : Sum
  Add_77142 : Sum
  Add_fff2e : Sum
  Constant_-1_54429 : Constant  Value=-1
  Constant_-1_950ae : Constant  Value=-1
  Constant_-1_d1a3b : Constant  Value=-1
  Constant_-2.0_b6484 : Constant  Value=-2.0
  Constant_T_1_89506 : Constant  Value=T_1
  Constant_T_1_e29f5 : Constant  Value=T_1
  Constant_T_2_c0e67 : Constant  Value=T_2
  Constant_T_3_bc104 : Constant  Value=T_3
  Constant_T_3_f2439 : Constant  Value=T_3
  Constant_T_4_f537a : Constant  Value=T_4
  Constant_T_w_cd1bd : Constant  Value=T_w
  Constant_T_w_db567 : Constant  Value=T_w
  Constant_f0_e11d4 : Constant  Value=f0
  Constant_pi_1bffd : Constant  Value=pi
  Divide_08592 : Product  Inputs=*/
  Divide_3963b : Product  Inputs=*/
  Divide_648b8 : Product  Inputs=*/
  Divide_7d10d : Product  Inputs=*/
  Divide_8775e : Product  Inputs=*/
  Divide_9d762 : Product  Inputs=*/
  Product_19037 : Product
  Product_49243 : Product
  Product_4ab01 : Product
  Product_7059c : Product
  Product_a3150 : Product
  Product_b756d : Product
  Product_ed4c1 : Product
  Blockout_d_Px_3_SG_D_3_2448a : Outport
  wires:
  State_Px_1_SG_D_3_ac5bc/1 -> Product_19037/2
  Constant_f0_e11d4/1 -> Product_a3150/2
  Constant_-2.0_b6484/1 -> Product_49243/1
  Add_36bb7/1 -> Divide_648b8/1
  Constant_pi_1bffd/1 -> Product_49243/2
  Product_49243/1 -> Product_a3150/1
  State_w_SG_D_3_60df7/1 -> Add_77142/2
  Constant_T_w_db567/1 -> Divide_3963b/2
  Constant_-1_54429/1 -> Product_19037/1
  Product_a3150/1 -> Add_77142/1
  Product_19037/1 -> Divide_3963b/1
  Add_77142/1 -> Divide_9d762/1
  Product_4ab01/1 -> Divide_7d10d/1
  Constant_T_w_cd1bd/1 -> Divide_9d762/2
  Divide_3963b/1 -> Add_4f5a0/1
  Divide_9d762/1 -> Add_4f5a0/2
  Constant_T_2_c0e67/1 -> Product_b756d/1
  Add_4f5a0/1 -> Product_b756d/2
  Constant_-1_d1a3b/1 -> Product_4ab01/1
  State_Px_2_SG_D_3_dd0dd/1 -> Product_4ab01/2
  State_Px_1_SG_D_3_57193/1 -> Add_36bb7/1
  Constant_T_3_f2439/1 -> Divide_08592/2
  Product_b756d/1 -> Add_36bb7/2
  Constant_T_1_e29f5/1 -> Divide_7d10d/2
  Add_fff2e/1 -> Product_7059c/2
  Constant_T_1_89506/1 -> Divide_648b8/2
  Divide_8775e/1 -> Add_3441e/2
  Divide_7d10d/1 -> Add_fff2e/1
  Divide_648b8/1 -> Add_fff2e/2
  Constant_T_4_f537a/1 -> Product_7059c/1
  Constant_-1_950ae/1 -> Product_ed4c1/1
  State_Px_3_SG_D_3_e3475/1 -> Product_ed4c1/2
  State_Px_2_SG_D_3_9be0b/1 -> Add_66dd9/1
  Product_7059c/1 -> Add_66dd9/2
  Product_ed4c1/1 -> Divide_08592/1
  Add_66dd9/1 -> Divide_8775e/1
  Constant_T_3_bc104/1 -> Divide_8775e/2
  Divide_08592/1 -> Add_3441e/1
  Add_3441e/1 -> Blockout_d_Px_3_SG_D_3_2448a/1
